simulink model "dcgidpimarycontrol"  (R2016b)
settings: Solver=VariableStepAuto  StartTime=0.0  StopTime=50  RelTol=1e-3
libraries: powerlib x62, simulink x12, powerlib_meascontrol x4
settings Model: Creator=ede  LastModifiedBy=jte-aar

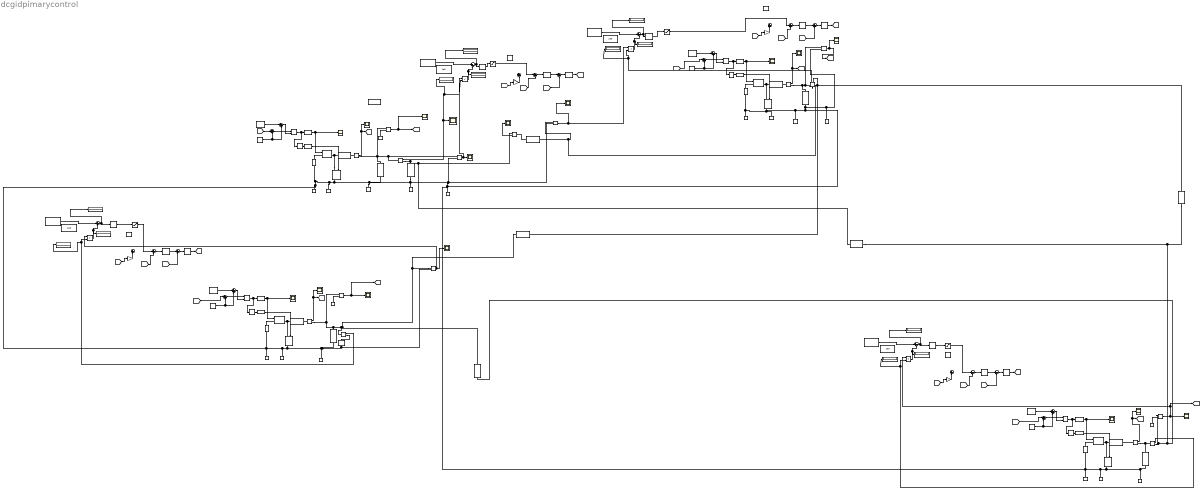
== system dcgidpimarycontrol ==
  Constant1 : Constant  Value=0.2944*1800*1e6
  Constant10 : Constant  Value=0.2222*1800*1e6
  Constant{5,9,11,16} (4 alike) : Constant  Value=1000
  Constant{2,6,12,14} (4 alike) : Constant  Value=1e5
  Constant13 : Constant  Value=0.0906*1800*1e6
  Constant{3,7..8,15} (4 alike) : Constant
  Constant4 : Constant  Value=0.3333*1800e6
  Current Measurement{1..9} (9 alike) : powerlib/Measurements/Current Measurement  PhasorSimulation=off  OutputType=Complex  PSBequivalent=0
  DC Voltage Source{1..4} (4 alike) : powerlib/Electrical Sources/DC Voltage Source  Amplitude=7e3  Measurements=None
  Data Type Conversion{1..8} (8 alike) : DataTypeConversion  OutDataTypeStr=double
  Display{,1..11} (12 alike) : Display
  Gain{1..4} (4 alike) : Gain  Gain=0.001
  Ideal Switch{1..2,5,7} (4 alike) : powerlib/Power Electronics/Ideal Switch  Ron=0.00000000005  Lon=0  IC=0  Rs=1e5  Cs=inf  Measurements=on
  Ideal Switch{3..4,6,8} (4 alike) : powerlib/Power Electronics/Ideal Switch  Ron=0.001  Lon=0  IC=0  Rs=1e5  Cs=inf  Measurements=on
  Logical Operator{1..4} (4 alike) : Logic  Operator=NOT  AllPortsSameDT=off  OutDataTypeStr=boolean
  Neutral{1..18} (18 alike) : powerlib/Elements/Neutral  LConnTagsString=a  NodeNumber=10
  PID Controller{,4,6,9} (4 alike) : simulink/Continuous/PID Controller  Controller=PID  TimeDomain=Continuous-time  SampleTime=-1  IntegratorMethod=Forward Euler  FilterMethod=Forward Euler  Form=Parallel  UseFilter=on  ControllerParametersSource=internal  P=0.01  I=1000  D=0.1  N=100  InitialConditionSource=internal  InitialConditionForIntegrator=0  InitialConditionForFilter=0  ExternalReset=none  LimitOutput=off  UpperSaturationLimit=inf  LowerSaturationLimit=-inf  LinearizeAsGain=on  AntiWindupMode=none  Kb=1  TrackingMode=off  Kt=1  PParamMin=[]  PParamMax=[]  IParamMin=[]  IParamMax=[]  DParamMin=[]  DParamMax=[]  NParamMin=[]  NParamMax=[]  KbParamMin=[]  KbParamMax=[]  KtParamMin=[]  KtParamMax=[]  POutMin=[]  POutMax=[]  IOutMin=[]  IOutMax=[]  DOutMin=[]  DOutMax=[]  NOutMin=[]  NOutMax=[]  KbOutMin=[]  KbOutMax=[]  KtOutMin=[]  KtOutMax=[]  IntegratorOutMin=[]  IntegratorOutMax=[]  FilterOutMin=[]  FilterOutMax=[]  SumOutMin=[]  SumOutMax=[]  SumI1OutMin=[]  SumI1OutMax=[]  SumI2OutMin=[]  SumI2OutMax=[]  SumI3OutMin=[]  SumI3OutMax=[]  SumDOutMin=[]  SumDOutMax=[]  SaturationOutMin=[]  SaturationOutMax=[]  IntegratorContinuousStateAttributes=''  IntegratorStateMustResolveToSignalObject=off  IntegratorRTWStateStorageClass=Auto  FilterContinuousStateAttributes=''  FilterStateMustResolveToSignalObject=off  FilterRTWStateStorageClass=Auto  DifferentiatorICPrevScaledInput=0  DifferentiatorOutMin=[]  DifferentiatorOutMax=[]
  PID Controller{1,3,8,11} (4 alike) : simulink/Continuous/PID Controller  Controller=PID  TimeDomain=Continuous-time  SampleTime=-1  IntegratorMethod=Forward Euler  FilterMethod=Forward Euler  Form=Parallel  UseFilter=on  ControllerParametersSource=internal  P=1.3e-5  I=1e-8  D=1e-10  N=100  InitialConditionSource=internal  InitialConditionForIntegrator=0  InitialConditionForFilter=0  ExternalReset=none  LimitOutput=off  UpperSaturationLimit=inf  LowerSaturationLimit=-inf  LinearizeAsGain=on  AntiWindupMode=none  Kb=1  TrackingMode=off  Kt=1  PParamMin=[]  PParamMax=[]  IParamMin=[]  IParamMax=[]  DParamMin=[]  DParamMax=[]  NParamMin=[]  NParamMax=[]  KbParamMin=[]  KbParamMax=[]  KtParamMin=[]  KtParamMax=[]  POutMin=[]  POutMax=[]  IOutMin=[]  IOutMax=[]  DOutMin=[]  DOutMax=[]  NOutMin=[]  NOutMax=[]  KbOutMin=[]  KbOutMax=[]  KtOutMin=[]  KtOutMax=[]  IntegratorOutMin=[]  IntegratorOutMax=[]  FilterOutMin=[]  FilterOutMax=[]  SumOutMin=[]  SumOutMax=[]  SumI1OutMin=[]  SumI1OutMax=[]  SumI2OutMin=[]  SumI2OutMax=[]  SumI3OutMin=[]  SumI3OutMax=[]  SumDOutMin=[]  SumDOutMax=[]  SaturationOutMin=[]  SaturationOutMax=[]  IntegratorContinuousStateAttributes=''  IntegratorStateMustResolveToSignalObject=off  IntegratorRTWStateStorageClass=Auto  FilterContinuousStateAttributes=''  FilterStateMustResolveToSignalObject=off  FilterRTWStateStorageClass=Auto  DifferentiatorICPrevScaledInput=0  DifferentiatorOutMin=[]  DifferentiatorOutMax=[]
  PID Controller{2,5,7,10} (4 alike) : simulink/Continuous/PID Controller  Controller=PID  TimeDomain=Continuous-time  SampleTime=-1  IntegratorMethod=Forward Euler  FilterMethod=Forward Euler  Form=Parallel  UseFilter=on  ControllerParametersSource=internal  P=0.01  I=10000  D=0.1  N=100  InitialConditionSource=internal  InitialConditionForIntegrator=0  InitialConditionForFilter=0  ExternalReset=none  LimitOutput=off  UpperSaturationLimit=inf  LowerSaturationLimit=-inf  LinearizeAsGain=on  AntiWindupMode=none  Kb=1  TrackingMode=off  Kt=1  PParamMin=[]  PParamMax=[]  IParamMin=[]  IParamMax=[]  DParamMin=[]  DParamMax=[]  NParamMin=[]  NParamMax=[]  KbParamMin=[]  KbParamMax=[]  KtParamMin=[]  KtParamMax=[]  POutMin=[]  POutMax=[]  IOutMin=[]  IOutMax=[]  DOutMin=[]  DOutMax=[]  NOutMin=[]  NOutMax=[]  KbOutMin=[]  KbOutMax=[]  KtOutMin=[]  KtOutMax=[]  IntegratorOutMin=[]  IntegratorOutMax=[]  FilterOutMin=[]  FilterOutMax=[]  SumOutMin=[]  SumOutMax=[]  SumI1OutMin=[]  SumI1OutMax=[]  SumI2OutMin=[]  SumI2OutMax=[]  SumI3OutMin=[]  SumI3OutMax=[]  SumDOutMin=[]  SumDOutMax=[]  SaturationOutMin=[]  SaturationOutMax=[]  IntegratorContinuousStateAttributes=''  IntegratorStateMustResolveToSignalObject=off  IntegratorRTWStateStorageClass=Auto  FilterContinuousStateAttributes=''  FilterStateMustResolveToSignalObject=off  FilterRTWStateStorageClass=Auto  DifferentiatorICPrevScaledInput=0  DifferentiatorOutMin=[]  DifferentiatorOutMax=[]
  Product{,1..3} (4 alike) : Product
  Relational Operator{1..4} (4 alike) : RelationalOperator  OutDataTypeStr=boolean  RndMeth=Nearest
  Saturation{,1..3} (4 alike) : Saturate  UpperLimit=1100  LowerLimit=900
  Scope{1..14,17,19,21} (17 alike) : Scope
  Series RLC Branch1 : powerlib/Elements/Series RLC Branch  LConnTagsString=__new0  RConnTagsString=__new0  BranchType=R  Resistance=1000^2/(0.517*1800*1e6)  Inductance=1e-3  SetiL0=off  InitialCurrent=0  Capacitance=1e-6  Setx0=off  InitialVoltage=0  Measurements=None
  Series RLC Branch10 : powerlib/Elements/Series RLC Branch  LConnTagsString=__new0  RConnTagsString=__new0  BranchType=R  Resistance=.07692*5.5555e-4  Inductance=1e-3  SetiL0=off  InitialCurrent=0  Capacitance=1e-6  Setx0=off  InitialVoltage=0  Measurements=None
  Series RLC Branch{2,5,7,11} (4 alike) : powerlib/Elements/Series RLC Branch  LConnTagsString=__new0  RConnTagsString=__new0  BranchType=L  Resistance=1e-20  Inductance=0.5e-3  SetiL0=off  InitialCurrent=0  Capacitance=1e-6  Setx0=off  InitialVoltage=0  Measurements=None
  Series RLC Branch{3,6,8,12} (4 alike) : powerlib/Elements/Series RLC Branch  LConnTagsString=__new0  RConnTagsString=__new0  BranchType=RC  Resistance=0.001  Inductance=1e-3  SetiL0=off  InitialCurrent=0  Capacitance=500e-3  Setx0=off  InitialVoltage=0  Measurements=None
  Series RLC Branch13 : powerlib/Elements/Series RLC Branch  LConnTagsString=__new0  RConnTagsString=__new0  BranchType=R  Resistance=.0555*5.5555e-4  Inductance=1e-3  SetiL0=off  InitialCurrent=0  Capacitance=1e-6  Setx0=off  InitialVoltage=0  Measurements=None
  Series RLC Branch15 : powerlib/Elements/Series RLC Branch  LConnTagsString=__new0  RConnTagsString=__new0  BranchType=R  Resistance=.0769*5.5555e-4  Inductance=1e-3  SetiL0=off  InitialCurrent=0  Capacitance=1e-6  Setx0=off  InitialVoltage=0  Measurements=None
  Series RLC Branch18 : powerlib/Elements/Series RLC Branch  LConnTagsString=__new0  RConnTagsString=__new0  BranchType=R  Resistance=.0454545*5.5555e-4  Inductance=1e-3  SetiL0=off  InitialCurrent=0  Capacitance=1e-6  Setx0=off  InitialVoltage=0  Measurements=None
  Series RLC Branch4 : powerlib/Elements/Series RLC Branch  LConnTagsString=__new0  RConnTagsString=__new0  BranchType=R  Resistance=.0555*5.5555e-4  Inductance=1e-3  SetiL0=off  InitialCurrent=0  Capacitance=1e-6  Setx0=off  InitialVoltage=0  Measurements=None
  Series RLC Branch9 : powerlib/Elements/Series RLC Branch  LConnTagsString=__new0  RConnTagsString=__new0  BranchType=R  Resistance=1000^2/(0.417*1800*1e6)  Inductance=1e-3  SetiL0=off  InitialCurrent=0  Capacitance=1e-6  Setx0=off  InitialVoltage=0  Measurements=None
  Sum{,1,4..5,8..11,14..17,20..23} (16 alike) : Sum  Inputs=|+-
  Sum{2..3,6..7,12..13,18..19} (8 alike) : Sum  Inputs=|++
  Triangle Generator{1..4} (4 alike) : powerlib_meascontrol/Pulse & Signal Generators/Triangle Generator  Freq=2e3  Phase=0  Ts=0
  Voltage Measurement{,1..6} (7 alike) : powerlib/Measurements/Voltage Measurement  PhasorSimulation=off  OutputType=Complex  PSBequivalent=0
  powergui : powerlib/powergui  Priority=1  SimulationMode=Discrete  SolverType=Tustin/Backward Euler (TBE)  SampleTime=1e-5  frequency=60  SPID=off  DisableSnubberDevices=off  DisableRonSwitches=off  DisableVfSwitches=off  SwTol=0  DisplayEquations=off  Interpol=off  ExternalGateDelay=off  methode=off  Ts=0  FunctionMessages=off  echomessages=off  HookPort=off  EnableUseOfTLC=off  x0status=blocks  frequencyindice=0  Pbase=100e6  ErrMax=1e-4  Iterations=50  UnitsV=kV  UnitsW=MW  buscounter=0  RestoreLinks=warning  ResistiveCurrentMeasurement=off  Frange=[10000:2:30000]  Ylog=on  Xlog=on  ShowGrid=on  save=on  variable=ZData  structure=Voltage  ZoomFFT=off  StartTime=0.05  cycles=1  DisplayStyle=1  fundamental=50  FreqAxis=off  MaxFrequency=6000  frequencyindicesteady=1  RmsSteady=1  display=off
  wires:
  Constant7/1 -> Sum2/2, Sum3/2
  Sum3/1 -> Relational Operator3/1
  [D1] -> Sum3/1
  Relational Operator3/1 -> Logical Operator1/1, Data Type Conversion4/1
  Data Type Conversion4/1 -> Scope19/1, Ideal Switch2/1
  Sum2/1 -> Relational Operator3/2
  Logical Operator1/1 -> Data Type Conversion5/1
  Data Type Conversion5/1 -> Ideal Switch3/1
  Current Measurement1/1 -> Scope17/1, [IL1]
  Voltage Measurement4/1 -> [VC1], Scope21/1
  Triangle Generator1/1 -> Sum2/1
  Sum1/1 -> PID Controller/1
  Gain4/1 -> Sum/2
  PID Controller/1 -> Sum8/1
  Sum8/1 -> PID Controller2/1
  PID Controller2/1 -> [D1]
  [VC1] -> Sum1/2
  [IL1] -> Gain4/1
  Product/1 -> Sum4/2, Display3/1
  Sum4/1 -> PID Controller1/1, Display/1
  [IL1] -> Sum8/2
  Current Measurement2/1 -> Scope2/1, Display1/1, Product/2
  Voltage Measurement1/1 -> Product/1, Scope1/1
  Constant1/1 -> Sum4/1
  Product1/1 -> Sum5/2, Display5/1
  Sum5/1 -> PID Controller3/1, Display2/1
  Voltage Measurement2/1 -> Product1/1, Scope3/1
  Constant4/1 -> Sum5/1
  Constant3/1 -> Sum6/2, Sum7/2
  Sum7/1 -> Relational Operator1/1
  [D2] -> Sum7/1
  Relational Operator1/1 -> Logical Operator2/1, Data Type Conversion1/1
  Data Type Conversion1/1 -> Scope5/1, Ideal Switch1/1
  Sum6/1 -> Relational Operator1/2
  Logical Operator2/1 -> Data Type Conversion2/1
  Data Type Conversion2/1 -> Ideal Switch4/1
  Current Measurement3/1 -> Scope4/1, [IL2]
  Triangle Generator2/1 -> Sum6/1
  Sum10/1 -> PID Controller4/1
  Gain1/1 -> Sum9/2
  PID Controller4/1 -> Sum11/1
  Sum11/1 -> PID Controller5/1
  PID Controller5/1 -> [D2]
  [VC2] -> Sum10/2
  [IL1] -> Gain1/1
  [IL2] -> Sum11/2
  Voltage Measurement/1 -> Scope9/1, [VC2]
  PID Controller3/1 -> Saturation1/1
  Constant8/1 -> Sum12/2, Sum13/2
  Sum13/1 -> Relational Operator2/1
  [D3] -> Sum13/1
  Relational Operator2/1 -> Logical Operator3/1, Data Type Conversion3/1
  Data Type Conversion3/1 -> Scope7/1, Ideal Switch5/1
  Sum12/1 -> Relational Operator2/2
  Logical Operator3/1 -> Data Type Conversion6/1
  Data Type Conversion6/1 -> Ideal Switch6/1
  Current Measurement5/1 -> Scope6/1, [IL3]
  Voltage Measurement3/1 -> Scope8/1, [VC3]
  Triangle Generator3/1 -> Sum12/1
  Sum14/1 -> PID Controller6/1
  Gain2/1 -> Sum16/2
  PID Controller6/1 -> Sum15/1
  Sum15/1 -> PID Controller7/1
  PID Controller7/1 -> [D3]
  [VC3] -> Sum14/2
  [IL1] -> Gain2/1
  [IL3] -> Sum15/2
  Product2/1 -> Sum17/2, Display8/1
  Sum17/1 -> PID Controller8/1, Display6/1
  Voltage Measurement5/1 -> Product2/1, Scope10/1
  Constant10/1 -> Sum17/1
  PID Controller8/1 -> Saturation3/1
  Constant15/1 -> Sum18/2, Sum19/2
  Sum19/1 -> Relational Operator4/1
  [D4] -> Sum19/1
  Relational Operator4/1 -> Logical Operator4/1, Data Type Conversion7/1
  Data Type Conversion7/1 -> Scope12/1, Ideal Switch7/1
  Sum18/1 -> Relational Operator4/2
  Logical Operator4/1 -> Data Type Conversion8/1
  Data Type Conversion8/1 -> Ideal Switch8/1
  Current Measurement7/1 -> Scope11/1, [IL4]
  Triangle Generator4/1 -> Sum18/1
  Sum20/1 -> PID Controller9/1
  Gain3/1 -> Sum22/2
  PID Controller9/1 -> Sum21/1
  Sum21/1 -> PID Controller10/1
  PID Controller10/1 -> [D4]
  [VC4] -> Sum20/2
  [IL4] -> Gain3/1
  [IL4] -> Sum21/2
  Product3/1 -> Sum23/2, Display11/1
  Sum23/1 -> PID Controller11/1, Display9/1
  Voltage Measurement6/1 -> Scope13/1, Product3/1, [VC4]
  Constant13/1 -> Sum23/1
  PID Controller11/1 -> Saturation2/1
  Current Measurement6/1 -> Display7/1, Product2/2
  Current Measurement8/1 -> Display10/1, Product3/2
  Current Measurement9/1 -> Display4/1, Product1/2
  Current Measurement4/1 -> Scope14/1
  PID Controller1/1 -> Saturation/1
  Saturation/1 -> Sum1/1
  Saturation1/1 -> Sum10/1
  Saturation2/1 -> Sum20/1
  Saturation3/1 -> Sum14/1
  connections:
  Ideal Switch3/LConn1 -- Series RLC Branch2/LConn1 -- Ideal Switch2/RConn1
  Voltage Measurement1/LConn1 -- Current Measurement2/LConn1 -- Series RLC Branch3/LConn1 -- Current Measurement1/RConn1 -- Voltage Measurement4/LConn1
  Ideal Switch2/LConn1 -- DC Voltage Source1/RConn1
  Current Measurement1/LConn1 -- Series RLC Branch2/RConn1
  Neutral18/LConn1 -- Ideal Switch8/RConn1 -- Neutral9/LConn1 -- Neutral1/LConn1 -- DC Voltage Source2/LConn1 -- Neutral8/LConn1 -- Ideal Switch4/RConn1 -- Voltage Measurement/LConn2 -- Neutral10/LConn1 -- Series RLC Branch6/RConn1 -- Voltage Measurement1/LConn2 -- Series RLC Branch1/RConn1 -- Neutral4/LConn1 -- Neutral6/LConn1 -- Neutral3/LConn1 -- Neutral5/LConn1 -- Voltage Measurement5/LConn2 -- Series RLC Branch9/RConn1 -- Series RLC Branch8/RConn1 -- Neutral11/LConn1 -- Neutral14/LConn1 -- Neutral13/LConn1 -- DC Voltage Source3/LConn1 -- Ideal Switch6/RConn1 -- DC Voltage Source1/LConn1 -- Ideal Switch3/RConn1 -- Series RLC Branch3/RConn1 -- Voltage Measurement2/LConn2 -- Neutral2/LConn1 -- Series RLC Branch12/RConn1 -- Neutral15/LConn1 -- Neutral17/LConn1 -- DC Voltage Source4/LConn1
  Voltage Measurement4/LConn2 -- Neutral7/LConn1
  Series RLC Branch4/RConn1 -- Current Measurement4/LConn1
  Current Measurement2/RConn1 -- Current Measurement4/RConn1 -- Series RLC Branch13/RConn1 -- Series RLC Branch1/LConn1
  Ideal Switch1/RConn1 -- Ideal Switch4/LConn1 -- Series RLC Branch5/LConn1
  Current Measurement3/LConn1 -- Series RLC Branch5/RConn1
  Ideal Switch1/LConn1 -- DC Voltage Source2/RConn1
  Ideal Switch5/RConn1 -- Ideal Switch6/LConn1 -- Series RLC Branch7/LConn1
  Current Measurement5/RConn1 -- Series RLC Branch8/LConn1 -- Current Measurement6/LConn1 -- Voltage Measurement5/LConn1 -- Series RLC Branch10/RConn1 -- Series RLC Branch18/LConn1 -- Voltage Measurement3/LConn1
  Current Measurement5/LConn1 -- Series RLC Branch7/RConn1
  Voltage Measurement3/LConn2 -- Neutral12/LConn1
  Ideal Switch5/LConn1 -- DC Voltage Source3/RConn1
  Voltage Measurement2/LConn1 -- Series RLC Branch15/RConn1 -- Current Measurement9/RConn1 -- Series RLC Branch10/LConn1 -- Series RLC Branch4/LConn1
  Ideal Switch7/RConn1 -- Ideal Switch8/LConn1 -- Series RLC Branch11/LConn1
  Voltage Measurement6/LConn1 -- Series RLC Branch15/LConn1 -- Series RLC Branch13/LConn1 -- Series RLC Branch18/RConn1 -- Current Measurement8/RConn1
  Ideal Switch7/LConn1 -- DC Voltage Source4/RConn1
  Voltage Measurement6/LConn2 -- Neutral16/LConn1
  Current Measurement7/LConn1 -- Series RLC Branch11/RConn1
  Current Measurement7/RConn1 -- Current Measurement8/LConn1 -- Series RLC Branch12/LConn1
  Current Measurement6/RConn1 -- Series RLC Branch9/LConn1
  Series RLC Branch6/LConn1 -- Current Measurement9/LConn1 -- Voltage Measurement/LConn1 -- Current Measurement3/RConn1
